simulink model "UWOC_Control_Model"  (R2024b)
settings: Solver=VariableStepAuto  StartTime=0.0  StopTime=50  RelTol=1e-3
undefined symbols (not defined in the file): A, K_lqr, prev_P_k, prev_u_k_ekf, prev_x_hat, Q_ekf, Q_sys, R_ekf, R_sys, u_k_lqr, x1_0
libraries: sharedTrackingLibrary x1, slpidlib x1
settings Model: Creator=grays  LastModifiedBy=tim
settings DebuggingCC: UnderSpecifiedDimensionMsg=warning

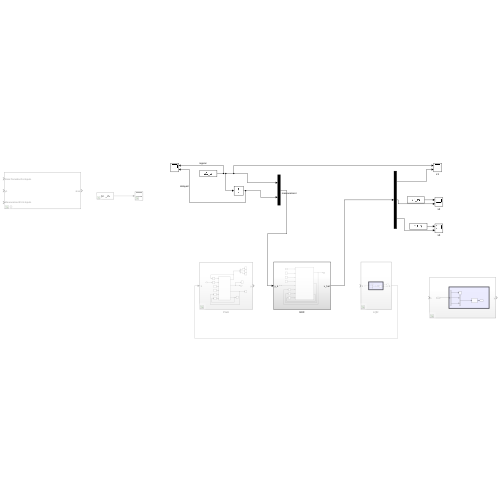
[thumbnail: Simulink's stored preview of the top-level diagram]
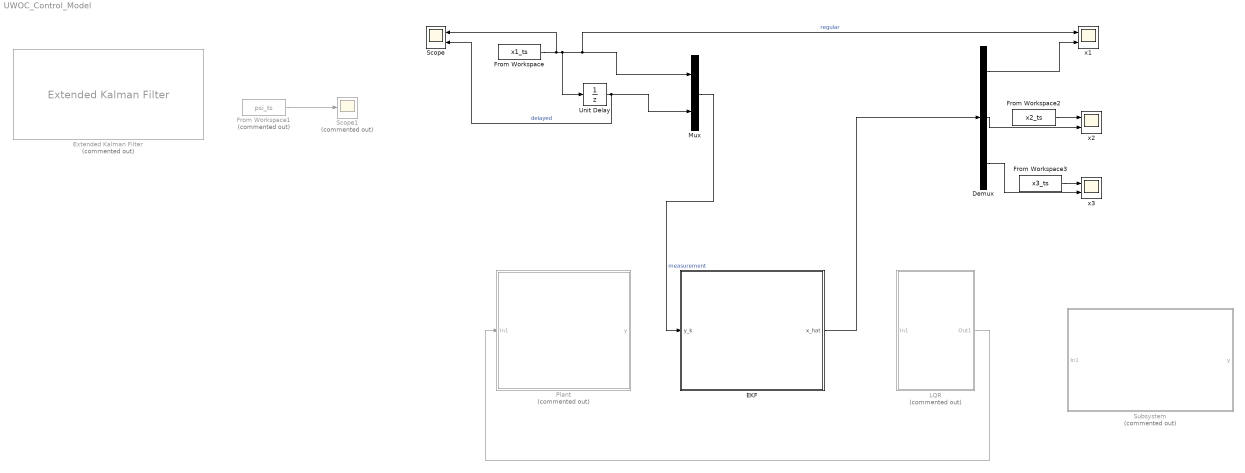
== system UWOC_Control_Model ==
  Demux : Demux  Outputs=3
  EKF : Subsystem
  Extended Kalman Filter : sharedTrackingLibrary/Extended Kalman Filter  Commented=on  StateTransitionFcn=0  HasStateTransitionJacobianFcn=off  HasAdditiveProcessNoise=Additive  ProcessNoise=Q_ekf  HasTimeVaryingProcessNoise=off  HasStateTransitionFcnExtraArgument=1  InitialState=[5; 2; 3]  InitialStateCovariance=1  MeasurementFcn1=y_hat_measurementFcn  HasMeasurementJacobianFcn1=off  HasMeasurementEnablePort1=off  HasAdditiveMeasurementNoise1=Additive  MeasurementNoise1=[1, 0; 0, 1]  HasTimeVaryingMeasurementNoise1=off  HasMeasurementFcnExtraArgument1=1  HasMeasurementWrapping1=off  MeasurementFcn2=myMeasurementFcn  HasMeasurementJacobianFcn2=off  HasMeasurementEnablePort2=off  HasAdditiveMeasurementNoise2=Additive  MeasurementNoise2=1  HasTimeVaryingMeasurementNoise2=off  HasMeasurementFcnExtraArgument2=0  HasMeasurementWrapping2=off  MeasurementFcn3=myMeasurementFcn  HasMeasurementJacobianFcn3=off  HasMeasurementEnablePort3=off  HasAdditiveMeasurementNoise3=Additive  MeasurementNoise3=1  HasTimeVaryingMeasurementNoise3=off  HasMeasurementFcnExtraArgument3=0  HasMeasurementWrapping3=off  MeasurementFcn4=myMeasurementFcn  HasMeasurementJacobianFcn4=off  HasMeasurementEnablePort4=off  HasAdditiveMeasurementNoise4=Additive  MeasurementNoise4=1  HasTimeVaryingMeasurementNoise4=off  HasMeasurementFcnExtraArgument4=0  HasMeasurementWrapping4=off  MeasurementFcn5=myMeasurementFcn  HasMeasurementJacobianFcn5=off  HasMeasurementEnablePort5=off  HasAdditiveMeasurementNoise5=Additive  MeasurementNoise5=1  HasTimeVaryingMeasurementNoise5=off  HasMeasurementFcnExtraArgument5=0  HasMeasurementWrapping5=off  EnableMultirate=off  StateTransitionFcnSampleTime=1  MeasurementFcn1SampleTime=1  MeasurementFcn2SampleTime=1  MeasurementFcn3SampleTime=1  MeasurementFcn4SampleTime=1  MeasurementFcn5SampleTime=1  UseCurrentEstimator=on  OutputStateCovariance=off  DataType=double  SampleTime=1  NumberOfMeasurements=1
  From Workspace : FromWorkspace  VariableName=x1_ts  SampleTime=0.1
  From Workspace1 : FromWorkspace  Commented=on  VariableName=psi_ts  SampleTime=0.01
  From Workspace2 : FromWorkspace  VariableName=x2_ts  SampleTime=0.1
  From Workspace3 : FromWorkspace  VariableName=x3_ts  SampleTime=0.1
  "LQR " : Subsystem  Commented=on
  Mux : Mux  Inputs=2
  Plant : Subsystem  Commented=on
  Scope : Scope  NumInputPorts=2
  Scope1 : Scope  Commented=on
  Subsystem : Subsystem  Commented=on
  Unit Delay : UnitDelay  InitialCondition=x1_0  SampleTime=-1  HasFrameUpgradeWarning=on
  x1 : Scope  NumInputPorts=2
  x2 : Scope  NumInputPorts=2
  x3 : Scope  NumInputPorts=2
  wires:
  From Workspace1/1 -> Scope1/1
  Demux/3 -> x3/2
  Demux/2 -> x2/2
  Demux/1 -> x1/2
  From Workspace3/1 -> x3/1
  From Workspace2/1 -> x2/1
  From Workspace/1 -> x1/1, Mux/1, Unit Delay/1, Scope/1  "regular"
  Unit Delay/1 -> Scope/2, Mux/2  "delayed"
  Mux/1 -> EKF/1(y_k)  "measurement"
  EKF/1(x_hat) -> Demux/1
  "LQR "/1(Out1) -> Plant/1(In1)

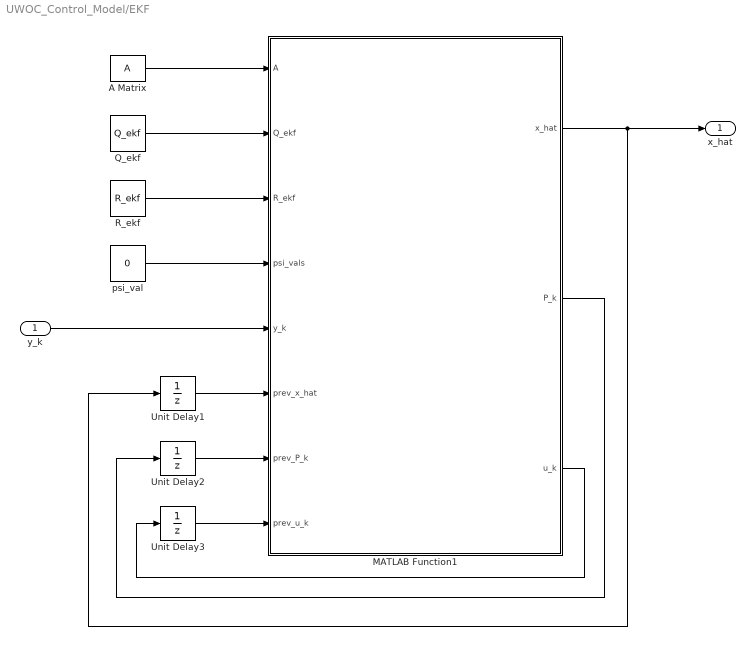
== system UWOC_Control_Model/EKF ==
  y_k : Inport
  A Matrix : Constant  Value=A
  MATLAB Function1 : MATLAB Function  TreatAsAtomicUnit=on
  Q_ekf : Constant  Value=Q_ekf
  R_ekf : Constant  Value=R_ekf
  Unit Delay1 : UnitDelay  InitialCondition=prev_x_hat  SampleTime=0.1  HasFrameUpgradeWarning=on
  Unit Delay2 : UnitDelay  InitialCondition=prev_P_k  SampleTime=0.1  HasFrameUpgradeWarning=on
  Unit Delay3 : UnitDelay  InitialCondition=prev_u_k_ekf  SampleTime=0.1  HasFrameUpgradeWarning=on
  psi_val : Constant  Value=0
  x_hat : Outport
  wires:
  MATLAB Function1/3(u_k) -> Unit Delay3/1
  MATLAB Function1/2(P_k) -> Unit Delay2/1
  Unit Delay3/1 -> MATLAB Function1/8(prev_u_k)
  MATLAB Function1/1(x_hat) -> x_hat/1, Unit Delay1/1
  A Matrix/1 -> MATLAB Function1/1(A)
  Unit Delay2/1 -> MATLAB Function1/7(prev_P_k)
  Unit Delay1/1 -> MATLAB Function1/6(prev_x_hat)
  Q_ekf/1 -> MATLAB Function1/2(Q_ekf)
  R_ekf/1 -> MATLAB Function1/3(R_ekf)
  psi_val/1 -> MATLAB Function1/4(psi_vals)
  y_k/1 -> MATLAB Function1/5(y_k)

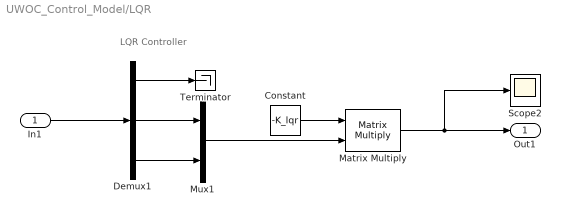
== system UWOC_Control_Model/LQR  ==
  note: LQR Controller
  In1 : Inport
  Constant : Constant  Value=-K_lqr  VectorParams1D=off
  Demux1 : Demux  Outputs=3
  Matrix Multiply : Product  Multiplication=Matrix(*)
  Mux1 : Mux  Inputs=2
  Scope2 : Scope
  Terminator : Terminator
  Out1 : Outport
  wires:
  Constant/1 -> Matrix Multiply/1
  Matrix Multiply/1 -> Out1/1, Scope2/1
  Demux1/1 -> Terminator/1
  Demux1/2 -> Mux1/1
  In1/1 -> Demux1/1
  Mux1/1 -> Matrix Multiply/2
  Demux1/3 -> Mux1/2

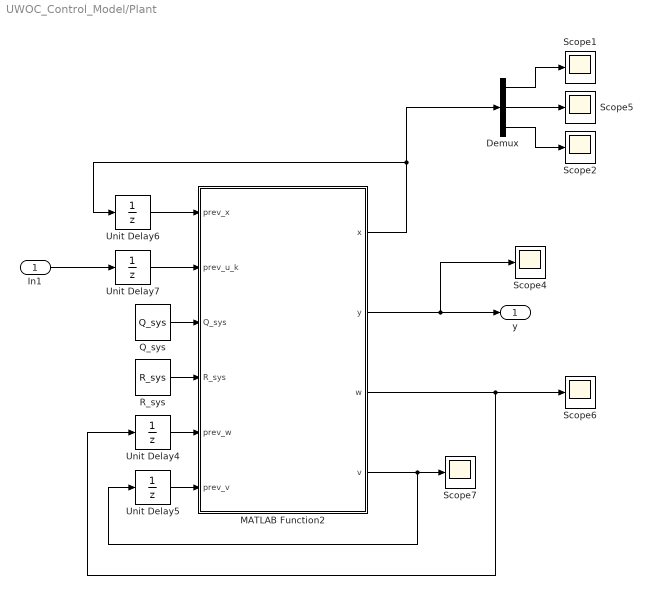
== system UWOC_Control_Model/Plant ==
  In1 : Inport
  Demux : Demux  Outputs=3
  MATLAB Function2 : MATLAB Function  TreatAsAtomicUnit=on
  Q_sys : Constant  Value=Q_sys  VectorParams1D=off
  R_sys : Constant  Value=R_sys  VectorParams1D=off
  Scope{1..2,4..7} (6 alike) : Scope
  Unit Delay4 : UnitDelay  InitialCondition=[0, 0, 0]  SampleTime=-1  HasFrameUpgradeWarning=on
  Unit Delay5 : UnitDelay  SampleTime=-1  HasFrameUpgradeWarning=on
  Unit Delay6 : UnitDelay  InitialCondition=[5, 2, 3]  SampleTime=-1  HasFrameUpgradeWarning=on
  Unit Delay7 : UnitDelay  InitialCondition=u_k_lqr  SampleTime=-1  HasFrameUpgradeWarning=on
  y : Outport
  wires:
  Unit Delay7/1 -> MATLAB Function2/2(prev_u_k)
  MATLAB Function2/3(w) -> Scope6/1, Unit Delay4/1
  Unit Delay6/1 -> MATLAB Function2/1(prev_x)
  Unit Delay5/1 -> MATLAB Function2/6(prev_v)
  MATLAB Function2/2(y) -> Scope4/1, y/1
  MATLAB Function2/4(v) -> Scope7/1, Unit Delay5/1
  MATLAB Function2/1(x) -> Demux/1, Unit Delay6/1
  In1/1 -> Unit Delay7/1
  Unit Delay4/1 -> MATLAB Function2/5(prev_w)
  R_sys/1 -> MATLAB Function2/4(R_sys)
  Q_sys/1 -> MATLAB Function2/3(Q_sys)
  Demux/2 -> Scope5/1
  Demux/1 -> Scope1/1
  Demux/3 -> Scope2/1

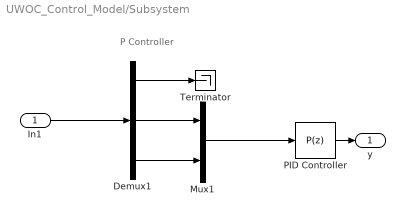
== system UWOC_Control_Model/Subsystem ==
  note: P Controller
  In1 : Inport
  Demux1 : Demux  Outputs=3
  Mux1 : Mux  Inputs=2
  PID Controller : slpidlib/PID Controller  Controller=P  Form=Parallel  TimeDomain=Discrete-time  UseExternalTs=off  SampleTime=-1  IntegratorMethod=Forward Euler  FilterMethod=Forward Euler  ControllerParametersSource=internal  P=[1, 1]  I=1  UseKiTs=off  D=0  UseExternalDerivativeSource=off  N=100  UseFilter=on  TunerSelectOption=Transfer Function Based (PID Tuner App)  InitialConditionSource=internal  InitialConditionForIntegrator=0  InitialConditionForFilter=0  DifferentiatorICPrevScaledInput=0  ExternalReset=none  TrackingMode=off  Kt=1  LimitOutput=off  SatLimitsSource=internal  UpperSaturationLimit=inf  LowerSaturationLimit=-inf  LinearizeAsGain=on  AntiWindupMode=none  Kb=1  LimitIntegrator=off  UpperIntegratorSaturationLimit=inf  LowerIntegratorSaturationLimit=-inf  POutMin=[]  POutMax=[]  IOutMin=[]  IOutMax=[]  DOutMin=[]  DOutMax=[]  NOutMin=[]  NOutMax=[]  SumOutMin=[]  SumOutMax=[]  SaturationOutMin=[]  SaturationOutMax=[]  PParamMin=[]  PParamMax=[]  IParamMin=[]  IParamMax=[]  DParamMin=[]  DParamMax=[]  NParamMin=[]  NParamMax=[]  KbParamMin=[]  KbParamMax=[]  KtParamMin=[]  KtParamMax=[]  KbOutMin=[]  KbOutMax=[]  KtOutMin=[]  KtOutMax=[]  IntegratorOutMin=[]  IntegratorOutMax=[]  FilterOutMin=[]  FilterOutMax=[]  SumI1OutMin=[]  SumI1OutMax=[]  SumI2OutMin=[]  SumI2OutMax=[]  SumI3OutMin=[]  SumI3OutMax=[]  SumI4OutMin=[]  SumI4OutMax=[]  SumDOutMin=[]  SumDOutMax=[]  DifferentiatorOutMin=[]  DifferentiatorOutMax=[]  FilterDiffOutCoefMin=[]  FilterDiffOutCoefMax=[]  ReciprocalOutMin=[]  ReciprocalOutMax=[]  SumDenOutMin=[]  SumDenOutMax=[]  SumNumOutMin=[]  SumNumOutMax=[]  DivideOutMin=[]  DivideOutMax=[]  UdiffTsProdOutMin=[]  UdiffTsProdOutMax=[]  NTsProdOutMin=[]  NTsProdOutMax=[]  UintegralTsProdOutMin=[]  UintegralTsProdOutMax=[]  UngainTsProdOutMin=[]  UngainTsProdOutMax=[]  ClampingZeroOutDataTypeStr=Inherit: Inherit via back propagation  ClampingZeroOutMin=[]  ClampingZeroOutMax=[]  FilterDenConstantOutDataTypeStr=Inherit: Inherit via back propagation  FilterDenConstantOutMin=[]  FilterDenConstantOutMax=[]  PCopyOutDataTypeStr=Inherit: Inherit via back propagation  PCopyOutMin=[]  PCopyOutMax=[]  NCopyOutDataTypeStr=Inherit: Inherit via back propagation  NCopyOutMin=[]  NCopyOutMax=[]  IntegratorContinuousStateAttributes=''  IntegratorStateMustResolveToSignalObject=off  IntegratorRTWStateStorageClass=Auto  FilterContinuousStateAttributes=''  FilterStateMustResolveToSignalObject=off  FilterRTWStateStorageClass=Auto  ParallelPVariant=InternalParameters  IdealPVariant=Disabled  IVariant=Disabled  DVariant=Disabled  IntegratorVariant=Disabled  SatVariant=Disabled  AWVariant=Disabled  PCopyVariant=Disabled  TRVariant=Disabled  FdbkBlocksVariant=Forward  IdealPFdbkVariant=Disabled  SatFdbkVariant=Disabled  DerivativeFilterVariant=Disabled  NVariant=Disabled  NCopyVariant=Disabled_SignalSpec  FilterICVariant=Disabled  IntegratorICVariant=Disabled  ExternalResetVariant=Disabled  TRSumVariant=Passthrough  SumFdbkVariant=Disabled  SumVariant=Passthrough_P  TsampFilterVariant=InternalTs  TsampNgainVariant=Passthrough  TsampIntegralVariant=Disabled_SignalSpec  ExternalSaturationOutDataTypeStr=Inherit: Same as second input  DerivativeSourceVariant=Disabled  PreIntVariant=InternalPreInt
  Terminator : Terminator
  y : Outport
  wires:
  Mux1/1 -> PID Controller/1
  Demux1/3 -> Mux1/2
  Demux1/1 -> Terminator/1
  Demux1/2 -> Mux1/1
  PID Controller/1 -> y/1
  In1/1 -> Demux1/1

== matlab function UWOC_Control_Model/EKF/MATLAB Function1 ==
  data: A input; x_hat output; Q_ekf input; R_ekf input; psi_vals input; y_k input; prev_x_hat input; prev_P_k input; prev_u_k input; P_k output; u_k output
function [x_hat, P_k, u_k]= ekf(A, Q_ekf, R_ekf, psi_vals, y_k, prev_x_hat, prev_P_k, prev_u_k)



x_hat = [prev_x_hat(1); prev_x_hat(2) + prev_x_hat(3); prev_x_hat(3) + prev_u_k];

P_k = A * prev_P_k* A' + Q_ekf;


% Work Needed to Compute Kalman Gain

%prev_u_k = -G(1) * prev_x_hat(2) - G(2) * prev_x_hat(3);

% Output Meaurements

%y_k = [x1_ts.Data(i); x1_ts.Data(i-1)];
%disp('y_k')
%disp(y_k)

%y_hat_k = [x_hat(1) * cos(x_hat(2) + psi_vals(i)); prev_x_hat(1) * cos(prev_x_hat(2) + psi_vals(i-1))];

% New h
%h = [x_hat(1) * cosd(x_hat(2) + psi_vals(i));
%    x_hat(1) * cosd(x_hat(2) - x_hat(3) + prev_u_k + psi_vals(i-1))];

% New h no psi test
h = [x_hat(1) * cosd(x_hat(2) + psi_vals(1));
    x_hat(1) * cosd(x_hat(2) - x_hat(3) + prev_u_k + psi_vals(1))];



y_hat_k = h;
%disp('y_hat_k')
%disp(y_hat_k)

% New Jacobian
%C = [cosd(x_hat(2) + psi_vals(i)), -x_hat(1) * sind(x_hat(2) + psi_vals(i)), 0;
%    cosd(x_hat(2)-x_hat(3) + prev_u_k + psi_vals(i-1)), -x_hat(1) * sind(x_hat(2)-x_hat(3)+ prev_u_k + psi_vals(i-1)), x_hat(1) * sind(x_hat(2) - x_hat(3) + prev_u_k + psi_vals(i-1))];

% New Jacobian No psi test
C = [cosd(x_hat(2) + psi_vals(1)), -x_hat(1) * sind(x_hat(2) + psi_vals(1)), 0;
    cosd(x_hat(2)-x_hat(3) + prev_u_k + psi_vals(1)), -x_hat(1) * sind(x_hat(2)-x_hat(3)+ prev_u_k + psi_vals(1)), x_hat(1) * sind(x_hat(2) - x_hat(3) + prev_u_k + psi_vals(1))];


% Compute Kalman Gain
K_k = P_k * C' * ((C * P_k * C') + R_ekf)^-1;


% Compute the Estimate

x_hat = x_hat + K_k*(y_k - y_hat_k);

% Compute the Error Covariance

P_k = P_k - (K_k * C * P_k);

u_k = (-(0.1) * x_hat(2)) - ((0.4) * x_hat(3));

%prev_u_k = u_k;
%prev_x_hat = x_hat;
%prev_P_k = P_k;

end

== matlab function UWOC_Control_Model/Plant/MATLAB Function2 ==
  data: x output; prev_x input; y output; prev_u_k input; Q_sys input; R_sys input; prev_w input; prev_v input; w output; v output
function [x, y, w, v] = UWOC_System_fcn(prev_x, prev_u_k, Q_sys, R_sys, prev_w, prev_v)

% Noise Parameters
mu = 0;
w = Q_sys * randn(3,1) + mu;
v = R_sys * randn(1,1) + mu;



x1 = prev_x(1) + prev_w(1);
x2 = prev_x(2) + prev_x(3) + prev_w(2);
x3 = prev_x(3) + prev_u_k + prev_w(3);

y1 = x1*cosd(x2) + v;
y2 = prev_x(1) * cosd(prev_x(2)) + prev_v;

y = [y1; y2];
x = [x1; x2; x3];
